simulink model "Exp_5"  (R2021a)
settings: Solver=VariableStepAuto  StartTime=0.0  StopTime=2  RelTol=1e-3
libraries: spsSeriesRLCBranchLib x2, spsCurrentMeasurementLib x2, spsDiodeLib x2, spsDCVoltageSourceLib x1, spsIdealSwitchLib x1, spsMultimeterLib x1, spsStairGeneratorLib x1, spspowerguiLib x1
settings Model: Creator=HP  LastModifiedBy=DCL

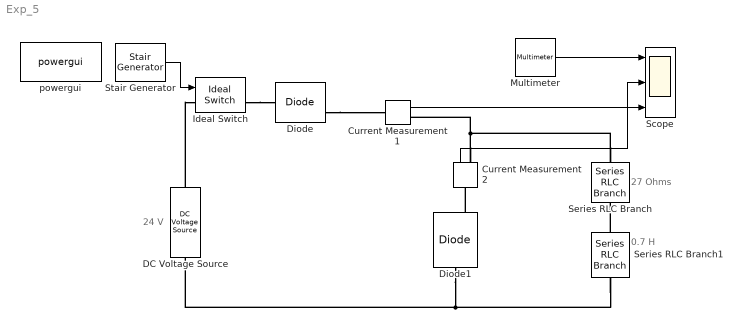
== system Exp_5 ==
  note: 27 Ohms
  note: 0.7 H
  note: 24 V
  " Series RLC Branch" : spsSeriesRLCBranchLib/Series RLC Branch  LConnTagsString=__new0  RConnTagsString=__new0  BranchType=R  Resistance=27  Inductance=2  SetiL0=off  InitialCurrent=0  Capacitance=1e-6  Setx0=off  InitialVoltage=0  Measurements=Branch voltage
  " Series RLC Branch1" : spsSeriesRLCBranchLib/Series RLC Branch  LConnTagsString=__new0  RConnTagsString=__new0  BranchType=L  Resistance=20  Inductance=0.7  SetiL0=off  InitialCurrent=0  Capacitance=0.5  Setx0=off  InitialVoltage=0  Measurements=None
  Current Measurement 1 : spsCurrentMeasurementLib/Current Measurement  PhasorSimulation=off  OutputType=Complex  PSBequivalent=0
  Current Measurement 2 : spsCurrentMeasurementLib/Current Measurement  PhasorSimulation=off  OutputType=Complex  PSBequivalent=0
  "DC Voltage Source " : spsDCVoltageSourceLib/DC Voltage Source  Amplitude=24  Measurements=None
  "Diode " : spsDiodeLib/Diode  Ron=0.001  Lon=0  Vf=0  IC=0  UseSnubber=0  Rs=500  Cs=250e-9  Measurements=on
  Diode1 : spsDiodeLib/Diode  Ron=0.001  Lon=0  Vf=0  IC=0  UseSnubber=0  Rs=500  Cs=250e-9  Measurements=on
  "Ideal Switch " : spsIdealSwitchLib/Ideal Switch  Ron=0.001  Lon=0  IC=0  Rs=1e5  Cs=inf  Measurements=on
  Multimeter : spsMultimeterLib/Multimeter  PhasorSimulation=off  OutputType=Complex  sel=1  L=1  Gain=1  yselected="{'Ub:  Series RLC Branch'};"  PSBOutputType=1  PSBequivalent=0  AxesSetting=[0,0.1,-100,100]  Display=1  SavedBlockNames=-11
  Scope : Scope  NumInputPorts=3
  "Stair Generator " : spsStairGeneratorLib/Stair Generator  t=[0, 1, 3, 3.5]  e=[1, -1, 2.5, 0]  Ts=0
  "powergui " : spspowerguiLib/powergui  Priority=1  SimulationMode=Continuous  SampleTime=50e-6  frequency=60  Iterations=50  frequencyindice=0  Pbase=100e6  ErrMax=1e-4  UnitsV=kV  UnitsW=MW  buscounter=0  FunctionMessages=off  echomessages=off  EnableUseOfTLC=off  CurrentSourceSwitches=off  DisableSnubberDevices=off  DisableRonSwitches=off  DisableVfSwitches=off  DisplayEquations=off  AutomaticDiscreteSolvers=off  SolverType=Tustin/Backward Euler (TBE)  Interpol=off  ExternalGateDelay=off  methode=off  Ts=100  x0status=blocks  SPID=on  SwTol=0  HookPort=off  NonlinearTolerance=1e-4  nMaxIteration=100  ContinueOnMaxIteration=off  RestoreLinks=warning  ResistiveCurrentMeasurement=off  Frange=[0:2:500]  Ylog=off  Xlog=on  ShowGrid=off  save=off  variable=ZData  structure=0  ZoomFFT=off  StartTime=0.0  cycles=1  DisplayStyle=1  fundamental=60  FreqAxis=off  MaxFrequency=1000  frequencyindicesteady=1  RmsSteady=1  display=off
  wires:
  "Stair Generator "/1 -> "Ideal Switch "/1
  Current Measurement 2/1 -> Scope/2
  Current Measurement 1/1 -> Scope/3
  Multimeter/1 -> Scope/1
  connections:
  "DC Voltage Source "/RConn1 -- "Ideal Switch "/LConn1
  "Ideal Switch "/RConn1 -- "Diode "/LConn1
  "Diode "/RConn1 -- Current Measurement 1/LConn1
  Diode1/RConn1 -- Current Measurement 2/LConn1
  Current Measurement 2/RConn1 -- Current Measurement 1/RConn1 -- " Series RLC Branch"/LConn1
  Diode1/LConn1 -- "DC Voltage Source "/LConn1 -- " Series RLC Branch1"/RConn1
  " Series RLC Branch1"/LConn1 -- " Series RLC Branch"/RConn1
